simulink model "trigger_02a"  (R2022a)
settings: Solver=VariableStepAuto  StartTime=0.0  StopTime=15  RelTol=1e-3
model workspace (MAT data in the model file):
  out_1 = 0
settings Model: Creator=FUGAZI  LastModifiedBy=FUGAZI

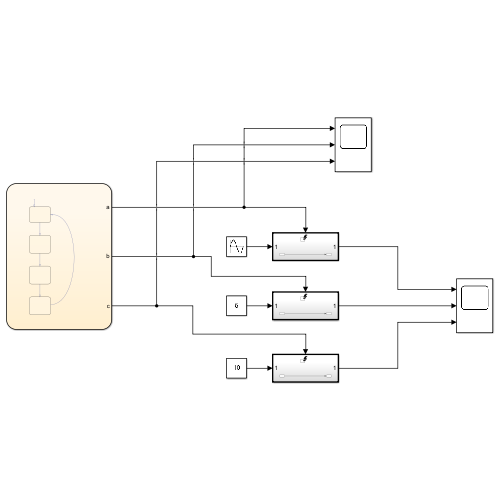
[thumbnail: Simulink's stored preview of the top-level diagram]
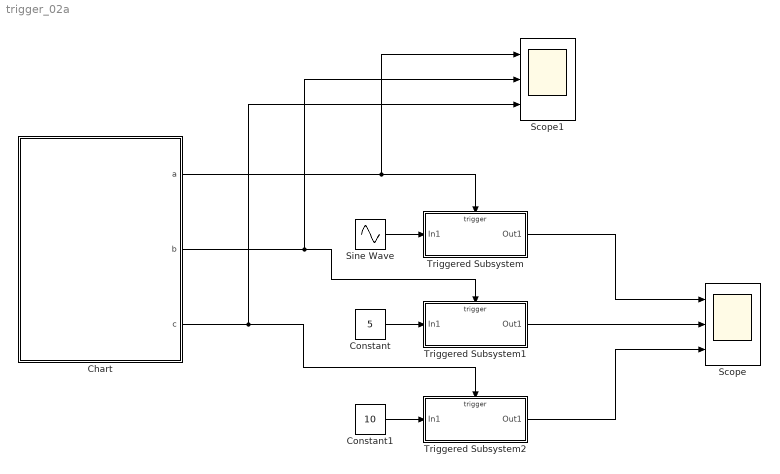
== system trigger_02a ==
  Chart : Stateflow chart  TreatAsAtomicUnit=on
      settings: PortSchema="{\"entries\":[{\"content\":{\"sides\":[{\"content\":{\"connectorIds\":[]},\"type\":\"ConnectorPlacement.EquallySpacedRectSide\",\"uuid\":\"b5cbc1c0-1000-46c0-8b8d-8ef2e8953df9\"},{\"content\":{\"connectorIds\":[\"Out1\",\"Out3\",\"Out2\"],\"side\":\"RIGHT\"},\"type\":\"ConnectorPlacement.EquallySpacedRectSide\",\"uuid\":\"5b481812-e16b-4050-8445-dc0ffc72983e\"},{\"content\":{\"connectorIds\":[],\"side\":\"TOP\"},\"type\":\"ConnectorPlacement.EquallySpacedRectSide\",\"uuid\":\"46103606-3d18-478c-b4ed-cdcad7e7e9e3\"}]},\"type\":\"ConnectorPlacement.EquallySpacedConnector\",\"uuid\":\"260628c0-7151-457e-9aaa-4ecee1bae499\"}],\"packageUris\":[\"http://schema.mathworks.com/mf0/Connector/R2020b\"],\"version\":\"1.0\"}"
  Constant : Constant  Value=5
  Constant1 : Constant  Value=10
  Scope : Scope  NumInputPorts=3
  Scope1 : Scope  NumInputPorts=3
  Sine Wave : Sin  SampleTime=0
  Triggered Subsystem : Subsystem  TreatAsAtomicUnit=on
  Triggered Subsystem1 : Subsystem  TreatAsAtomicUnit=on
  Triggered Subsystem2 : Subsystem  TreatAsAtomicUnit=on
  wires:
  Triggered Subsystem/1(Out1) -> Scope/1
  Chart/1(a) -> Triggered Subsystem/Trigger, Scope1/1
  Chart/3(b) -> Triggered Subsystem1/Trigger, Scope1/2
  Chart/2(c) -> Triggered Subsystem2/Trigger, Scope1/3
  Sine Wave/1 -> Triggered Subsystem/1(In1)
  Constant/1 -> Triggered Subsystem1/1(In1)
  Constant1/1 -> Triggered Subsystem2/1(In1)
  Triggered Subsystem1/1(Out1) -> Scope/2
  Triggered Subsystem2/1(Out1) -> Scope/3

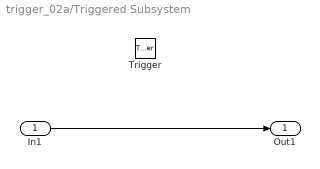
== system trigger_02a/Triggered Subsystem ==
  In1 : Inport
  Trigger : TriggerPort  VariantControl=(inherit)
  Out1 : Outport
  wires:
  In1/1 -> Out1/1

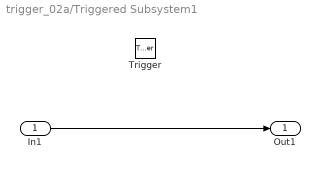
== system trigger_02a/Triggered Subsystem1 ==
  In1 : Inport
  Trigger : TriggerPort  VariantControl=(inherit)
  Out1 : Outport
  wires:
  In1/1 -> Out1/1

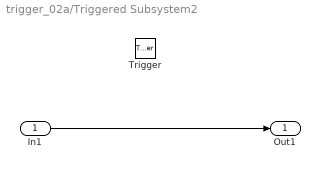
== system trigger_02a/Triggered Subsystem2 ==
  In1 : Inport
  Trigger : TriggerPort  VariantControl=(inherit)
  Out1 : Outport
  wires:
  In1/1 -> Out1/1

== stateflow chart trigger_02a/Chart ==
  state start
    a = 0;
    b = 0;
    c = 0;
  state step_1
    a = 1;
    b = 0;
    c = 0;
  state step_2
    a = 0;
    b = 1;
    c = 0;
  state step_3
    a = 0;
    b = 0;
    c = 1;
  (default) -> start
  step_3 -> start : after(2,sec)
  start -> step_1 : [after(2,sec)]
  step_1 -> step_2 : [after(2,sec)]
  step_2 -> step_3 : [after(2,sec)]
  data: a output; c output; b output
